simulink model "smtp_task"  (Simulink 3.00)
undefined symbols (not defined in the file): Device, My, REX
libraries: stringlib x6, mathlib x3, speclib x1

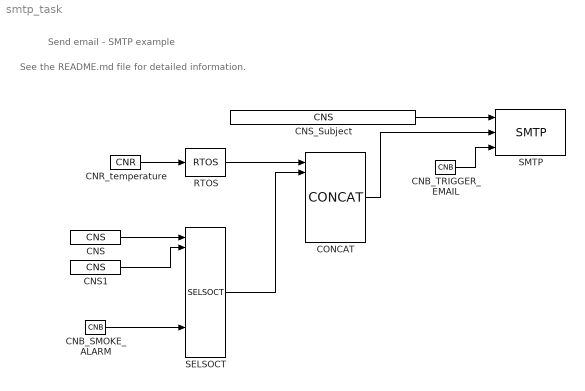
== system smtp_task ==
  note: See the README.md file for detailed information.
  note: Send email - SMTP example
  CNB_SMOKE_ALARM : mathlib/CNB  YCN=on
  CNB_TRIGGER_EMAIL : mathlib/CNB  YCN=off
  CNR_temperature : mathlib/CNR  ycn=21.7
  CNS : stringlib/CNS  scv=inactive  nmax=0
  CNS1 : stringlib/CNS  scv=active  nmax=0
  CNS_Subject : stringlib/CNS  scv=Message from REX  nmax=0
  CONCAT : stringlib/CONCAT  ptrn=Hi there,\nthis is a message from REX. Temperature is %1 and the smoke sensor is %2.\nHave a nice day!  nmax=0
  RTOS : stringlib/RTOS  prec=5  mode=1: best fit
  SELSOCT : stringlib/SELSOCT  BINF=on  nmax=0
  SMTP : speclib/SMTP  server=smtp.gmail.com  to=recipient@domain.com  from=youraccount@gmail.com  tls=3: TLS  user=youraccount  password=yourpassword  domain=My-REX-Device  auth=1: Login  certificate=""  VERIFY=off  timeout=20  BLOCKING=off  nmax=256  datamax=1024
  wires:
  CNB_SMOKE_ALARM/1 -> SELSOCT/10
  CNB_TRIGGER_EMAIL/1 -> SMTP/3
  CNR_temperature/1 -> RTOS/1
  CNS/1 -> SELSOCT/1
  CNS1/1 -> SELSOCT/2
  CNS_Subject/1 -> SMTP/1
  CONCAT/1 -> SMTP/2
  RTOS/1 -> CONCAT/1
  SELSOCT/1 -> CONCAT/2
